simulink model "Robot_Model_2"  (R2022b)
settings: Solver=FixedStepAuto  StartTime=0.0  StopTime=120  FixedStep=Sample_T  RelTol=1e-3
values from neighbouring files (symbols this model uses):
  B = 0.4    [Model_script.m]
  Dynamics_on = 0    [Model_script.m]
  Ka = 1    [Model_script.m]
  l = 0.6    [Model_script.m]
  r = 0.05    [Model_script.m]
  Slip_on = 0    [Model_script.m]
  Slip_time = 0.25    [Model_script.m]
  Tau = 0.4    [Model_script.m]
libraries: simulink x2
settings Model: Creator=pl130  LastModifiedBy=pl130

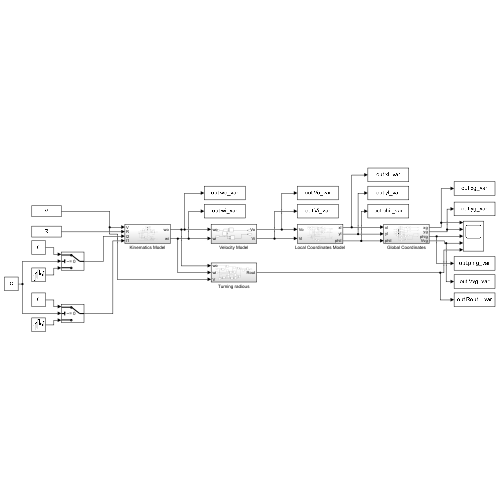
[thumbnail: Simulink's stored preview of the top-level diagram]
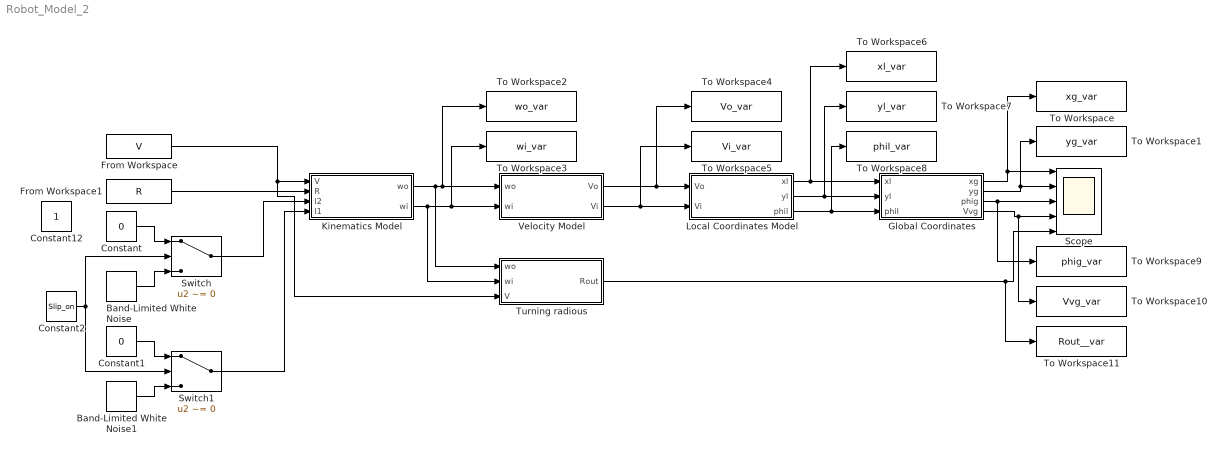
== system Robot_Model_2 ==
  Band-Limited White Noise : simulink/Sources/Band-Limited White Noise  Cov=Slip_power  Ts=Slip_time  seed=[23341]
  Band-Limited White Noise1 : simulink/Sources/Band-Limited White Noise  Cov=Slip_power  Ts=Slip_time  seed=[54352]
  Constant : Constant  Value=0
  Constant1 : Constant  Value=0
  Constant2 : Constant  Value=Slip_on
  From Workspace : FromWorkspace  VariableName=V
  From Workspace1 : FromWorkspace  VariableName=R
  Global Coordinates : Subsystem
  Kinematics Model : Subsystem
  Local Coordinates Model : Subsystem
  Scope : Scope  NumInputPorts=5
  Switch : Switch  Criteria=u2 ~= 0  SaturateOnIntegerOverflow=off  InputSameDT=off
  Switch1 : Switch  Criteria=u2 ~= 0  SaturateOnIntegerOverflow=off  InputSameDT=off
  To Workspace : ToWorkspace  VariableName=xg_var  SampleTime=-1
  To Workspace1 : ToWorkspace  VariableName=yg_var  SampleTime=-1
  To Workspace10 : ToWorkspace  VariableName=Vvg_var  SampleTime=-1
  To Workspace11 : ToWorkspace  VariableName=Rout__var  SampleTime=-1
  To Workspace2 : ToWorkspace  VariableName=wo_var  SampleTime=-1
  To Workspace3 : ToWorkspace  VariableName=wi_var  SampleTime=-1
  To Workspace4 : ToWorkspace  VariableName=Vo_var  SampleTime=-1
  To Workspace5 : ToWorkspace  VariableName=Vi_var  SampleTime=-1
  To Workspace6 : ToWorkspace  VariableName=xl_var  SampleTime=-1
  To Workspace7 : ToWorkspace  VariableName=yl_var  SampleTime=-1
  To Workspace8 : ToWorkspace  VariableName=phil_var  SampleTime=-1
  To Workspace9 : ToWorkspace  VariableName=phig_var  SampleTime=-1
  Turning radious : Subsystem
  Velocity Model : Subsystem
  Constant12 : Constant  IOType=siggen
  wires:
  Kinematics Model/1(wo) -> Turning radious/1(wo), To Workspace2/1, Velocity Model/1(wo)
  Kinematics Model/2(wi) -> Turning radious/2(wi), To Workspace3/1, Velocity Model/2(wi)
  Local Coordinates Model/1(xl) -> To Workspace6/1, Global Coordinates/1(xl)
  Local Coordinates Model/2(yl) -> To Workspace7/1, Global Coordinates/2(yl)
  Local Coordinates Model/3(phil) -> To Workspace8/1, Global Coordinates/3(phil)
  Turning radious/1(Rout) -> To Workspace11/1, Scope/5
  From Workspace/1 -> Turning radious/3(V), Kinematics Model/1(V)
  Global Coordinates/1(xg) -> To Workspace/1, Scope/1
  Global Coordinates/2(yg) -> To Workspace1/1, Scope/2
  Global Coordinates/3(phig) -> Scope/3, To Workspace9/1
  Global Coordinates/4(Vvg) -> To Workspace10/1, Scope/4
  Velocity Model/1(Vo) -> To Workspace4/1, Local Coordinates Model/1(Vo)
  Velocity Model/2(Vi) -> To Workspace5/1, Local Coordinates Model/2(Vi)
  From Workspace1/1 -> Kinematics Model/2(R)
  Constant/1 -> Switch/1
  Constant1/1 -> Switch1/1
  Constant2/1 -> Switch/2, Switch1/2
  Band-Limited White Noise/1 -> Switch/3
  Band-Limited White Noise1/1 -> Switch1/3
  Switch/1 -> Kinematics Model/3(l2)
  Switch1/1 -> Kinematics Model/4(l1)

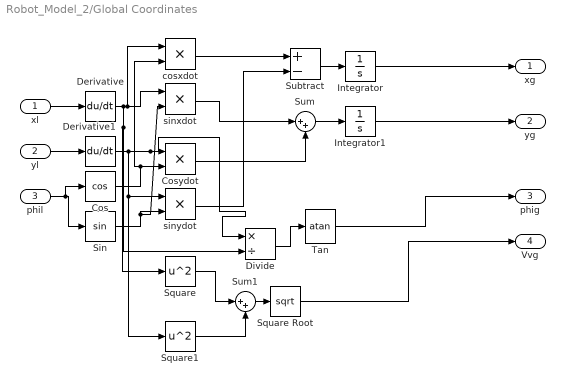
== system Robot_Model_2/Global Coordinates ==
  xl : Inport
  yl : Inport  Port=2
  phil : Inport  Port=3
  Cos : Trigonometry  Operator=cos
  Cosydot : Product
  Derivative : Derivative
  Derivative1 : Derivative
  Divide : Product  Inputs=*/
  Integrator : Integrator
  Integrator1 : Integrator
  Sin : Trigonometry
  Square : Math  Operator=square
  Square Root : Sqrt
  Square1 : Math  Operator=square
  Subtract : Sum  Inputs=+-
  Sum : Sum  Inputs=|++
  Sum1 : Sum  Inputs=|++
  Tan : Trigonometry  Operator=atan
  cosxdot : Product
  sinxdot : Product
  sinydot : Product
  xg : Outport
  yg : Outport  Port=2
  phig : Outport  Port=3
  Vvg : Outport  Port=4
  wires:
  xl/1 -> Derivative/1
  yl/1 -> Derivative1/1
  phil/1 -> Cos/1, Sin/1
  Derivative1/1 -> Divide/1, Cosydot/1, Square1/1, sinydot/1
  Cos/1 -> Cosydot/2, cosxdot/2
  Sin/1 -> sinxdot/2, sinydot/2
  Derivative/1 -> Divide/2, Square/1, cosxdot/1, sinxdot/1
  cosxdot/1 -> Subtract/1
  sinydot/1 -> Subtract/2
  Subtract/1 -> Integrator/1
  Integrator/1 -> xg/1
  Sum/1 -> Integrator1/1
  sinxdot/1 -> Sum/1
  Cosydot/1 -> Sum/2
  Integrator1/1 -> yg/1
  Tan/1 -> phig/1
  Square/1 -> Sum1/1
  Square1/1 -> Sum1/2
  Square Root/1 -> Vvg/1
  Divide/1 -> Tan/1
  Sum1/1 -> Square Root/1

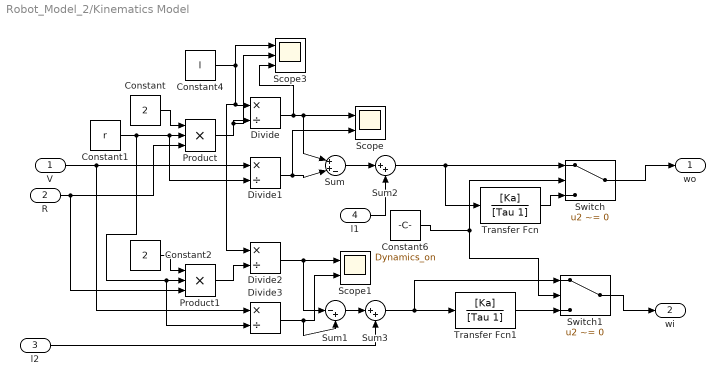
== system Robot_Model_2/Kinematics Model ==
  V : Inport
  R : Inport  Port=2
  l2 : Inport  Port=3
  l1 : Inport  Port=4
  Constant : Constant  Value=2
  Constant1 : Constant  Value=r
  Constant2 : Constant  Value=2
  Constant4 : Constant  Value=l
  Constant6 : Constant  Value=Dynamics_on
  Divide{,1..3} (4 alike) : Product  Inputs=*/
  Product : Product  Inputs=3
  Product1 : Product  Inputs=3
  Scope : Scope  NumInputPorts=2
  Scope1 : Scope  NumInputPorts=2
  Scope3 : Scope  NumInputPorts=3
  Sum : Sum  Inputs=|++-
  Sum1 : Sum  Inputs=|-+
  Sum2 : Sum  Inputs=|++
  Sum3 : Sum  Inputs=|++
  Switch : Switch  Criteria=u2 ~= 0  SaturateOnIntegerOverflow=off  InputSameDT=off
  Switch1 : Switch  Criteria=u2 ~= 0  SaturateOnIntegerOverflow=off  InputSameDT=off
  Transfer Fcn : TransferFcn  Numerator=[Ka]  Denominator=[Tau 1]
  Transfer Fcn1 : TransferFcn  Numerator=[Ka]  Denominator=[Tau 1]
  wo : Outport
  wi : Outport  Port=2
  wires:
  Constant/1 -> Product/1
  Constant1/1 -> Divide3/2, Product1/2, Divide1/2, Product/2
  Constant4/1 -> Divide2/1, Divide/1, Scope3/1
  Product/1 -> Scope3/2, Divide/2
  Divide/1 -> Scope3/3, Sum/1, Scope/1
  Divide1/1 -> Sum/2, Scope/2
  Divide3/1 -> Scope1/2, Sum1/2
  Product1/1 -> Divide2/2
  Divide2/1 -> Sum1/1, Scope1/1
  R/1 -> Product1/3, Product/3
  Constant2/1 -> Product1/1
  V/1 -> Divide1/1, Divide3/1
  Sum/1 -> Sum2/1
  Sum1/1 -> Sum3/1
  l2/1 -> Sum3/2
  l1/1 -> Sum2/2
  Transfer Fcn/1 -> Switch/3
  Constant6/1 -> Switch/2, Switch1/2
  Sum2/1 -> Transfer Fcn/1, Switch/1
  Sum3/1 -> Switch1/1, Transfer Fcn1/1
  Transfer Fcn1/1 -> Switch1/3
  Switch1/1 -> wi/1
  Switch/1 -> wo/1

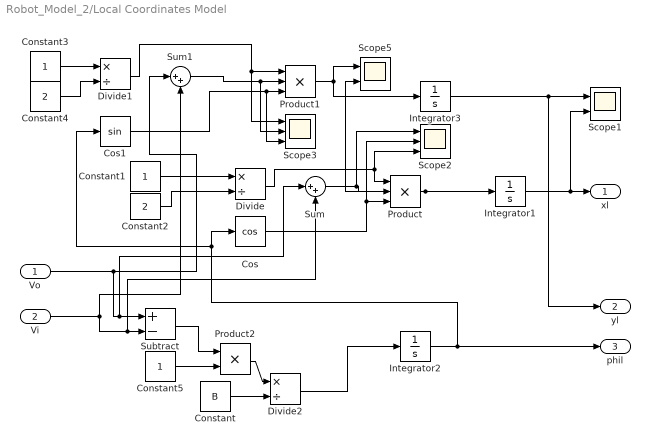
== system Robot_Model_2/Local Coordinates Model ==
  Vo : Inport
  Vi : Inport  Port=2
  Constant : Constant  Value=B
  Constant1 : Constant
  Constant2 : Constant  Value=2
  Constant3 : Constant
  Constant4 : Constant  Value=2
  Constant5 : Constant
  Cos : Trigonometry  Operator=cos
  Cos1 : Trigonometry
  Divide : Product  Inputs=*/
  Divide1 : Product  Inputs=*/
  Divide2 : Product  Inputs=*/
  Integrator1 : Integrator  InitialCondition=0.01
  Integrator2 : Integrator
  Integrator3 : Integrator  InitialCondition=0.01
  Product : Product  Inputs=3
  Product1 : Product  Inputs=3
  Product2 : Product
  Scope1 : Scope  NumInputPorts=2
  Scope2 : Scope  NumInputPorts=3
  Scope3 : Scope  NumInputPorts=3
  Scope5 : Scope  NumInputPorts=2
  Subtract : Sum  Inputs=+-
  Sum : Sum  Inputs=|++
  Sum1 : Sum  Inputs=|++
  xl : Outport
  yl : Outport  Port=2
  phil : Outport  Port=3
  wires:
  Constant/1 -> Divide2/2
  Subtract/1 -> Product2/1
  Constant1/1 -> Divide/1
  Constant2/1 -> Divide/2
  Divide/1 -> Product/1, Scope2/3
  Cos/1 -> Scope2/2, Product/3
  Product/1 -> Integrator1/1, Scope5/2
  Constant3/1 -> Divide1/1
  Divide1/1 -> Product1/1, Scope3/1
  Constant4/1 -> Divide1/2
  Vi/1 -> Sum1/2, Sum/2, Subtract/2
  Cos1/1 -> Scope3/3, Product1/3
  Vo/1 -> Sum1/1, Sum/1, Subtract/1
  Product1/1 -> Integrator3/1, Scope5/1
  Integrator2/1 -> Cos1/1, Cos/1, phil/1
  Sum1/1 -> Scope3/2, Product1/2
  Constant5/1 -> Product2/2
  Divide2/1 -> Integrator2/1
  Product2/1 -> Divide2/1
  Sum/1 -> Scope2/1, Product/2
  Integrator1/1 -> Scope1/2, xl/1
  Integrator3/1 -> yl/1, Scope1/1

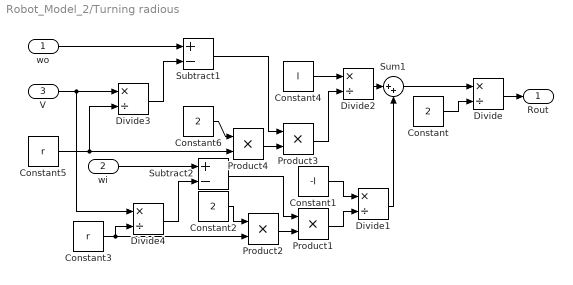
== system Robot_Model_2/Turning radious ==
  wo : Inport
  wi : Inport  Port=2
  V : Inport  Port=3
  Constant : Constant  Value=2
  Constant1 : Constant  Value=-l
  Constant2 : Constant  Value=2
  Constant3 : Constant  Value=r
  Constant4 : Constant  Value=l
  Constant5 : Constant  Value=r
  Constant6 : Constant  Value=2
  Divide{,1..4} (5 alike) : Product  Inputs=*/
  Product{1..4} (4 alike) : Product
  Subtract1 : Sum  Inputs=+-
  Subtract2 : Sum  Inputs=+-
  Sum1 : Sum  Inputs=|++
  Rout : Outport
  wires:
  Constant4/1 -> Divide2/1
  Product4/1 -> Product3/2
  Constant5/1 -> Divide3/2, Product4/2
  Constant6/1 -> Product4/1
  wo/1 -> Subtract1/1
  Divide3/1 -> Subtract1/2
  V/1 -> Divide4/1, Divide3/1
  Subtract1/1 -> Product3/1
  Product3/1 -> Divide2/2
  Divide2/1 -> Sum1/1
  Constant2/1 -> Product2/1
  wi/1 -> Subtract2/1
  Divide4/1 -> Subtract2/2
  Product2/1 -> Product1/2
  Product1/1 -> Divide1/2
  Constant1/1 -> Divide1/1
  Divide1/1 -> Sum1/2
  Subtract2/1 -> Product1/1
  Constant3/1 -> Divide4/2, Product2/2
  Sum1/1 -> Divide/1
  Constant/1 -> Divide/2
  Divide/1 -> Rout/1

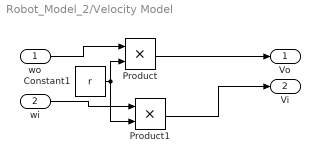
== system Robot_Model_2/Velocity Model ==
  wo : Inport
  wi : Inport  Port=2
  Constant1 : Constant  Value=r
  Product : Product
  Product1 : Product
  Vo : Outport
  Vi : Outport  Port=2
  wires:
  wo/1 -> Product/1
  Constant1/1 -> Product/2, Product1/2
  Product/1 -> Vo/1
  wi/1 -> Product1/1
  Product1/1 -> Vi/1
